simulink model "control_pos_6dof_conMI"  (R2023b)
settings: Solver=ode45  StartTime=0.0  StopTime=tsim  FixedStep=tstep  MaxStep=tstep
undefined symbols (not defined in the file): a0, a1, MI_Contr1, MI_Contr2, MI_Contr3, MI_Contr4, MI_Contr5, MI_Contr6, MI_motor1, MI_motor2, MI_motor3, MI_motor4, MI_motor5, MI_motor6, robot_params, sigbuilder_block, t_qeq_init, t_tr_init, tau_L, tr_ref
(part 6 of 10)

== matlab function control_pos_6dof_conMI/Controlador/Modelo dinámico ==
  data: robot_params input; robot_din output Bus: robot_din_bus size=1; q input size=[6,1]; dq input size=[6,1]
function robot_din = fcn(robot_params,q,dq)


% l1 = robot_params.l(1);
l2 = robot_params.l(2);
l3 = robot_params.l(3);
% l4 = robot_params.l(4);
% l5 = robot_params.l(5);
% l6 = robot_params.l(6);

lc1 = robot_params.lc(1);
lc2 = robot_params.lc(2);
lc3 = robot_params.lc(3);
% lc4 = robot_params.lc(4);
% lc5 = robot_params.lc(5);
% lc6 = robot_params.lc(6);

d1 = robot_params.d(1);
d2 = robot_params.d(2);
d3 = robot_params.d(3);
d4 = robot_params.d(4);
d5 = robot_params.d(5);
d6 = robot_params.d(6);

% dc1 = robot_params.dc(1);
% dc2 = robot_params.dc(2);
% dc3 = robot_params.dc(3);
dc4 = robot_params.dc(4);
dc5 = robot_params.dc(5);
dc6 = robot_params.dc(6);

m1 = robot_params.m(1);
m2 = robot_params.m(2);
m3 = robot_params.m(3);
m4 = robot_params.m(4);
m5 = robot_params.m(5);
m6 = robot_params.m(6);

%Posiciones angulares
% q1 = q(1);
q2 = q(2);
q3 = q(3);
q4 = q(4);
q5 = q(5);
% q6 = q(6);

%Velocidades angulares
dq1 = dq(1);
dq2 = dq(2);
dq3 = dq(3);
dq4 = dq(4);
dq5 = dq(5);
% dq6 = dq(6);

% Matriz de Inercia D
D = zeros(6,6);

D(1,1) = (d1*m1)/2 + (d2*m2)/2 + (d3*m3)/2 + (d4*m4)/2 + (d5*m5)/2 + (d6*m6)/2 + d4^2*m5 + d4^2*m6 + (d5^2*m6)/2 + dc4^2*m4 + (dc5^2*m5)/2 + (3*dc6^2*m6)/4 + (l2^2*m3)/2 + (l2^2*m4)/2 + (l2^2*m5)/2 + (l3^2*m4)/2 + (l2^2*m6)/2 + (l3^2*m5)/2 + (l3^2*m6)/2 + lc1^2*m1 + (lc2^2*m2)/2 + (lc3^2*m3)/2 - (dc6^2*m6*cos(2*q2 + 2*q3 + 2*q4 - 2*q5))/8 - (dc6^2*m6*cos(2*q2 + 2*q3 + 2*q4 + 2*q5))/8 - (d5^2*m6*cos(2*q2 + 2*q3 + 2*q4))/2 + (dc6^2*m6*cos(2*q5))/4 - (dc5^2*m5*cos(2*q2 + 2*q3 + 2*q4))/2 + (dc6^2*m6*cos(2*q2 + 2*q3 + 2*q4))/4 + (l2^2*m3*cos(2*q2))/2 + (l2^2*m4*cos(2*q2))/2 + (l2^2*m5*cos(2*q2))/2 + (l2^2*m6*cos(2*q2))/2 + (lc2^2*m2*cos(2*q2))/2 + (l3^2*m4*cos(2*q2 + 2*q3))/2 + (l3^2*m5*cos(2*q2 + 2*q3))/2 + (l3^2*m6*cos(2*q2 + 2*q3))/2 + (lc3^2*m3*cos(2*q2 + 2*q3))/2 + d5*l2*m6*sin(2*q2 + q3 + q4) + dc5*l2*m5*sin(2*q2 + q3 + q4) + (dc6*l2*m6*sin(q3 + q4 - q5))/2 + (d5*dc6*m6*cos(2*q2 + 2*q3 + 2*q4 + q5))/2 + d5*l2*m6*sin(q3 + q4) + dc5*l2*m5*sin(q3 + q4) - (dc6*l3*m6*sin(q4 + q5))/2 + (dc6*l3*m6*sin(2*q2 + 2*q3 + q4 - q5))/2 + 2*d4*dc6*m6*cos(q5) + l2*l3*m4*cos(q3) + l2*l3*m5*cos(q3) + l2*l3*m6*cos(q3) + l2*lc3*m3*cos(q3) + d5*l3*m6*sin(q4) + d5*l3*m6*sin(2*q2 + 2*q3 + q4) + dc5*l3*m5*sin(q4) + dc5*l3*m5*sin(2*q2 + 2*q3 + q4) - (dc6*l2*m6*sin(2*q2 + q3 + q4 + q5))/2 - (d5*dc6*m6*cos(2*q2 + 2*q3 + 2*q4 - q5))/2 + l2*l3*m4*cos(2*q2 + q3) + l2*l3*m5*cos(2*q2 + q3) + l2*l3*m6*cos(2*q2 + q3) + l2*lc3*m3*cos(2*q2 + q3) + (dc6*l3*m6*sin(q4 - q5))/2 - (dc6*l2*m6*sin(q3 + q4 + q5))/2 + (dc6*l2*m6*sin(2*q2 + q3 + q4 - q5))/2 - (dc6*l3*m6*sin(2*q2 + 2*q3 + q4 + q5))/2;
D(1,2) = (dc6^2*m6*cos(q2 + q3 + q4 - 2*q5))/4 - (dc6^2*m6*cos(q2 + q3 + q4 + 2*q5))/4 - (d4*dc6*m6*cos(q2 + q3 + q4 + q5))/2 + (d5*dc6*m6*cos(q2 + q3 + q4 + q5))/2 - (dc6*l3*m6*sin(q2 + q3 - q5))/2 - d4*l3*m5*sin(q2 + q3) - d4*l3*m6*sin(q2 + q3) - dc4*l3*m4*sin(q2 + q3) - (dc6*l2*m6*sin(q2 + q5))/2 + (d4*dc6*m6*cos(q2 + q3 + q4 - q5))/2 + (d5*dc6*m6*cos(q2 + q3 + q4 - q5))/2 - d4*l2*m5*sin(q2) - d4*l2*m6*sin(q2) - dc4*l2*m4*sin(q2) + d4*d5*m6*cos(q2 + q3 + q4) + d4*dc5*m5*cos(q2 + q3 + q4) - (dc6*l2*m6*sin(q2 - q5))/2 - (dc6*l3*m6*sin(q2 + q3 + q5))/2;
D(1,3) = (dc6^2*m6*cos(q2 + q3 + q4 - 2*q5))/4 - (dc6^2*m6*cos(q2 + q3 + q4 + 2*q5))/4 - (d4*dc6*m6*cos(q2 + q3 + q4 + q5))/2 + (d5*dc6*m6*cos(q2 + q3 + q4 + q5))/2 - (dc6*l3*m6*sin(q2 + q3 - q5))/2 - d4*l3*m5*sin(q2 + q3) - d4*l3*m6*sin(q2 + q3) - dc4*l3*m4*sin(q2 + q3) + (d4*dc6*m6*cos(q2 + q3 + q4 - q5))/2 + (d5*dc6*m6*cos(q2 + q3 + q4 - q5))/2 + d4*d5*m6*cos(q2 + q3 + q4) + d4*dc5*m5*cos(q2 + q3 + q4) - (dc6*l3*m6*sin(q2 + q3 + q5))/2;
D(1,4) = (dc6^2*m6*cos(q2 + q3 + q4 - 2*q5))/4 - (dc6^2*m6*cos(q2 + q3 + q4 + 2*q5))/4 - (d4*dc6*m6*cos(q2 + q3 + q4 + q5))/2 + (d5*dc6*m6*cos(q2 + q3 + q4 + q5))/2 + (d4*dc6*m6*cos(q2 + q3 + q4 - q5))/2 + (d5*dc6*m6*cos(q2 + q3 + q4 - q5))/2 + d4*d5*m6*cos(q2 + q3 + q4) + d4*dc5*m5*cos(q2 + q3 + q4);
D(1,5) = -(dc6*m6*(d4*cos(q2 + q3 + q4 + q5) + d5*cos(q2 + q3 + q4 + q5) + l3*sin(q2 + q3 - q5) - l2*sin(q2 + q5) + d4*cos(q2 + q3 + q4 - q5) - d5*cos(q2 + q3 + q4 - q5) + 2*dc6*cos(q2 + q3 + q4) + l2*sin(q2 - q5) - l3*sin(q2 + q3 + q5)))/2;
D(1,6) = 0;

D(2,1) = (dc6^2*m6*cos(q2 + q3 + q4 - 2*q5))/4 - (dc6^2*m6*cos(q2 + q3 + q4 + 2*q5))/4 - (d4*dc6*m6*cos(q2 + q3 + q4 + q5))/2 + (d5*dc6*m6*cos(q2 + q3 + q4 + q5))/2 - (dc6*l3*m6*sin(q2 + q3 - q5))/2 - d4*l3*m5*sin(q2 + q3) - d4*l3*m6*sin(q2 + q3) - dc4*l3*m4*sin(q2 + q3) - (dc6*l2*m6*sin(q2 + q5))/2 + (d4*dc6*m6*cos(q2 + q3 + q4 - q5))/2 + (d5*dc6*m6*cos(q2 + q3 + q4 - q5))/2 - d4*l2*m5*sin(q2) - d4*l2*m6*sin(q2) - dc4*l2*m4*sin(q2) + d4*d5*m6*cos(q2 + q3 + q4) + d4*dc5*m5*cos(q2 + q3 + q4) - (dc6*l2*m6*sin(q2 - q5))/2 - (dc6*l3*m6*sin(q2 + q3 + q5))/2;
D(2,2) = (d2*m2)/2 + (d3*m3)/2 + (d4*m4)/2 + (d5*m5)/2 + (d6*m6)/2 + d5^2*m6 + dc5^2*m5 + (dc6^2*m6)/2 + l2^2*m3 + l2^2*m4 + l2^2*m5 + l3^2*m4 + l2^2*m6 + l3^2*m5 + l3^2*m6 + lc2^2*m2 + lc3^2*m3 - (dc6^2*m6*cos(2*q5))/2 + 2*d5*l2*m6*sin(q3 + q4) + 2*dc5*l2*m5*sin(q3 + q4) + 2*l2*l3*m4*cos(q3) + 2*l2*l3*m5*cos(q3) + 2*l2*l3*m6*cos(q3) + 2*l2*lc3*m3*cos(q3) + 2*d5*l3*m6*sin(q4) + 2*dc5*l3*m5*sin(q4) - 2*dc6*l3*m6*cos(q4)*sin(q5) - 2*dc6*l2*m6*cos(q3)*cos(q4)*sin(q5) + 2*dc6*l2*m6*sin(q3)*sin(q4)*sin(q5);
D(2,3) = d5^2*m6 + dc5^2*m5 + (dc6^2*m6)/2 + l3^2*m4 + l3^2*m5 + l3^2*m6 + lc3^2*m3 - (dc6^2*m6*cos(2*q5))/2 + d5*l2*m6*sin(q3 + q4) + dc5*l2*m5*sin(q3 + q4) + l2*l3*m4*cos(q3) + l2*l3*m5*cos(q3) + l2*l3*m6*cos(q3) + l2*lc3*m3*cos(q3) + 2*d5*l3*m6*sin(q4) + 2*dc5*l3*m5*sin(q4) - 2*dc6*l3*m6*cos(q4)*sin(q5) - dc6*l2*m6*cos(q3)*cos(q4)*sin(q5) + dc6*l2*m6*sin(q3)*sin(q4)*sin(q5);
D(2,4) = d5^2*m6 + dc5^2*m5 + (dc6^2*m6)/2 - (dc6^2*m6*cos(2*q5))/2 + d5*l2*m6*sin(q3 + q4) + dc5*l2*m5*sin(q3 + q4) + d5*l3*m6*sin(q4) + dc5*l3*m5*sin(q4) - dc6*l3*m6*cos(q4)*sin(q5) - dc6*l2*m6*cos(q3)*cos(q4)*sin(q5) + dc6*l2*m6*sin(q3)*sin(q4)*sin(q5);
D(2,5) = -dc6*m6*cos(q5)*(d5 + l2*sin(q3 + q4) + l3*sin(q4));
D(2,6) = 0;

D(3,1) = (dc6^2*m6*cos(q2 + q3 + q4 - 2*q5))/4 - (dc6^2*m6*cos(q2 + q3 + q4 + 2*q5))/4 - (d4*dc6*m6*cos(q2 + q3 + q4 + q5))/2 + (d5*dc6*m6*cos(q2 + q3 + q4 + q5))/2 - (dc6*l3*m6*sin(q2 + q3 - q5))/2 - d4*l3*m5*sin(q2 + q3) - d4*l3*m6*sin(q2 + q3) - dc4*l3*m4*sin(q2 + q3) + (d4*dc6*m6*cos(q2 + q3 + q4 - q5))/2 + (d5*dc6*m6*cos(q2 + q3 + q4 - q5))/2 + d4*d5*m6*cos(q2 + q3 + q4) + d4*dc5*m5*cos(q2 + q3 + q4) - (dc6*l3*m6*sin(q2 + q3 + q5))/2;
D(3,2) = d5^2*m6 + dc5^2*m5 + (dc6^2*m6)/2 + l3^2*m4 + l3^2*m5 + l3^2*m6 + lc3^2*m3 - (dc6^2*m6*cos(2*q5))/2 + d5*l2*m6*sin(q3 + q4) + dc5*l2*m5*sin(q3 + q4) + l2*l3*m4*cos(q3) + l2*l3*m5*cos(q3) + l2*l3*m6*cos(q3) + l2*lc3*m3*cos(q3) + 2*d5*l3*m6*sin(q4) + 2*dc5*l3*m5*sin(q4) - 2*dc6*l3*m6*cos(q4)*sin(q5) - dc6*l2*m6*cos(q3)*cos(q4)*sin(q5) + dc6*l2*m6*sin(q3)*sin(q4)*sin(q5);
D(3,3) = (d3*m3)/2 + (d4*m4)/2 + (d5*m5)/2 + (d6*m6)/2 + d5^2*m6 + dc5^2*m5 + l3^2*m4 + l3^2*m5 + l3^2*m6 + lc3^2*m3 + dc6^2*m6*sin(q5)^2 + 2*d5*l3*m6*sin(q4) + 2*dc5*l3*m5*sin(q4) - 2*dc6*l3*m6*cos(q4)*sin(q5);
D(3,4) = d5^2*m6 + dc5^2*m5 + dc6^2*m6*sin(q5)^2 + d5*l3*m6*sin(q4) + dc5*l3*m5*sin(q4) - dc6*l3*m6*cos(q4)*sin(q5);
D(3,5) = -dc6*m6*cos(q5)*(d5 + l3*sin(q4));
D(3,6) = 0;

D(4,1) = (dc6^2*m6*cos(q2 + q3 + q4 - 2*q5))/4 - (dc6^2*m6*cos(q2 + q3 + q4 + 2*q5))/4 - (d4*dc6*m6*cos(q2 + q3 + q4 + q5))/2 + (d5*dc6*m6*cos(q2 + q3 + q4 + q5))/2 + (d4*dc6*m6*cos(q2 + q3 + q4 - q5))/2 + (d5*dc6*m6*cos(q2 + q3 + q4 - q5))/2 + d4*d5*m6*cos(q2 + q3 + q4) + d4*dc5*m5*cos(q2 + q3 + q4);
D(4,2) = d5^2*m6 + dc5^2*m5 + (dc6^2*m6)/2 - (dc6^2*m6*cos(2*q5))/2 + d5*l2*m6*sin(q3 + q4) + dc5*l2*m5*sin(q3 + q4) + d5*l3*m6*sin(q4) + dc5*l3*m5*sin(q4) - dc6*l3*m6*cos(q4)*sin(q5) - dc6*l2*m6*cos(q3)*cos(q4)*sin(q5) + dc6*l2*m6*sin(q3)*sin(q4)*sin(q5);
D(4,3) = d5^2*m6 + dc5^2*m5 + dc6^2*m6*sin(q5)^2 + d5*l3*m6*sin(q4) + dc5*l3*m5*sin(q4) - dc6*l3*m6*cos(q4)*sin(q5);
D(4,4) = (d4*m4)/2 + (d5*m5)/2 + (d6*m6)/2 + d5^2*m6 + dc5^2*m5 + dc6^2*m6 - dc6^2*m6*cos(q5)^2;
D(4,5) = -d5*dc6*m6*cos(q5);
D(4,6) = 0;

D(5,1) = -(dc6*m6*(d4*cos(q2 + q3 + q4 + q5) + d5*cos(q2 + q3 + q4 + q5) + l3*sin(q2 + q3 - q5) - l2*sin(q2 + q5) + d4*cos(q2 + q3 + q4 - q5) - d5*cos(q2 + q3 + q4 - q5) + 2*dc6*cos(q2 + q3 + q4) + l2*sin(q2 - q5) - l3*sin(q2 + q3 + q5)))/2;
D(5,2) = -dc6*m6*cos(q5)*(d5 + l2*sin(q3 + q4) + l3*sin(q4));
D(5,3) = -dc6*m6*cos(q5)*(d5 + l3*sin(q4));
D(5,4) = -d5*dc6*m6*cos(q5);
D(5,5) = (d5*m5)/2 + (d6*m6)/2 + dc6^2*m6;
D(5,6) = 0;

D(6,1) = 0;
D(6,2) = 0;
D(6,3) = 0;
D(6,4) = 0;
D(6,5) = 0;
D(6,6) = 1;

% Matriz de Coriollis C
C = zeros(6,6);

C(1,1) = 0;
C(1,2) = (dc6^2*dq1*m6*sin(2*q2 + 2*q3 + 2*q4 - 2*q5))/4 + (dc6^2*dq1*m6*sin(2*q2 + 2*q3 + 2*q4 + 2*q5))/4 + d5^2*dq1*m6*sin(2*q2 + 2*q3 + 2*q4) + dc5^2*dq1*m5*sin(2*q2 + 2*q3 + 2*q4) - (dc6^2*dq1*m6*sin(2*q2 + 2*q3 + 2*q4))/2 - dq1*l2^2*m3*sin(2*q2) - dq1*l2^2*m4*sin(2*q2) - dq1*l2^2*m5*sin(2*q2) - dq1*l2^2*m6*sin(2*q2) - dq1*lc2^2*m2*sin(2*q2) - dq1*l3^2*m4*sin(2*q2 + 2*q3) - dq1*l3^2*m5*sin(2*q2 + 2*q3) - dq1*l3^2*m6*sin(2*q2 + 2*q3) - dq1*lc3^2*m3*sin(2*q2 + 2*q3) - (dc6^2*dq2*m6*sin(q2 + q3 + q4 - 2*q5))/4 + (dc6^2*dq2*m6*sin(q2 + q3 + q4 + 2*q5))/4 - (dc6*dq2*l2*m6*cos(q2 - q5))/2 + d5*dc6*dq1*m6*sin(2*q2 + 2*q3 + 2*q4 - q5) - (dc6*dq2*l3*m6*cos(q2 + q3 + q5))/2 - 2*dq1*l2*l3*m4*sin(2*q2 + q3) - 2*dq1*l2*l3*m5*sin(2*q2 + q3) - 2*dq1*l2*l3*m6*sin(2*q2 + q3) - 2*dq1*l2*lc3*m3*sin(2*q2 + q3) - d4*d5*dq2*m6*sin(q2 + q3 + q4) - d4*dc5*dq2*m5*sin(q2 + q3 + q4) + dc6*dq1*l2*m6*cos(2*q2 + q3 + q4 - q5) - dc6*dq1*l3*m6*cos(2*q2 + 2*q3 + q4 + q5) + 2*d5*dq1*l2*m6*cos(2*q2 + q3 + q4) + 2*dc5*dq1*l2*m5*cos(2*q2 + q3 + q4) - (dc6*dq2*l3*m6*cos(q2 + q3 - q5))/2 + (d4*dc6*dq2*m6*sin(q2 + q3 + q4 + q5))/2 - (d5*dc6*dq2*m6*sin(q2 + q3 + q4 + q5))/2 - d4*dq2*l3*m5*cos(q2 + q3) - d4*dq2*l3*m6*cos(q2 + q3) - dc4*dq2*l3*m4*cos(q2 + q3) - (dc6*dq2*l2*m6*cos(q2 + q5))/2 + dc6*dq1*l3*m6*cos(2*q2 + 2*q3 + q4 - q5) - d5*dc6*dq1*m6*sin(2*q2 + 2*q3 + 2*q4 + q5) - d4*dq2*l2*m5*cos(q2) - d4*dq2*l2*m6*cos(q2) + 2*d5*dq1*l3*m6*cos(2*q2 + 2*q3 + q4) - dc4*dq2*l2*m4*cos(q2) + 2*dc5*dq1*l3*m5*cos(2*q2 + 2*q3 + q4) - dc6*dq1*l2*m6*cos(2*q2 + q3 + q4 + q5) - (d4*dc6*dq2*m6*sin(q2 + q3 + q4 - q5))/2 - (d5*dc6*dq2*m6*sin(q2 + q3 + q4 - q5))/2;
C(1,3) = (dc6^2*dq1*m6*sin(2*q2 + 2*q3 + 2*q4 - 2*q5))/4 + (dc6^2*dq1*m6*sin(2*q2 + 2*q3 + 2*q4 + 2*q5))/4 + d5^2*dq1*m6*sin(2*q2 + 2*q3 + 2*q4) + dc5^2*dq1*m5*sin(2*q2 + 2*q3 + 2*q4) - (dc6^2*dq1*m6*sin(2*q2 + 2*q3 + 2*q4))/2 - dq1*l3^2*m4*sin(2*q2 + 2*q3) - dq1*l3^2*m5*sin(2*q2 + 2*q3) - dq1*l3^2*m6*sin(2*q2 + 2*q3) - dq1*lc3^2*m3*sin(2*q2 + 2*q3) - (dc6^2*dq2*m6*sin(q2 + q3 + q4 - 2*q5))/2 + (dc6^2*dq2*m6*sin(q2 + q3 + q4 + 2*q5))/2 - (dc6^2*dq3*m6*sin(q2 + q3 + q4 - 2*q5))/4 + (dc6^2*dq3*m6*sin(q2 + q3 + q4 + 2*q5))/4 + d5*dc6*dq1*m6*sin(2*q2 + 2*q3 + 2*q4 - q5) - (dc6*dq1*l2*m6*cos(q3 + q4 + q5))/2 - dc6*dq2*l3*m6*cos(q2 + q3 + q5) - (dc6*dq3*l3*m6*cos(q2 + q3 + q5))/2 - dq1*l2*l3*m4*sin(2*q2 + q3) - dq1*l2*l3*m5*sin(2*q2 + q3) - dq1*l2*l3*m6*sin(2*q2 + q3) - dq1*l2*lc3*m3*sin(2*q2 + q3) - 2*d4*d5*dq2*m6*sin(q2 + q3 + q4) - d4*d5*dq3*m6*sin(q2 + q3 + q4) - 2*d4*dc5*dq2*m5*sin(q2 + q3 + q4) - d4*dc5*dq3*m5*sin(q2 + q3 + q4) + (dc6*dq1*l2*m6*cos(2*q2 + q3 + q4 - q5))/2 - dc6*dq1*l3*m6*cos(2*q2 + 2*q3 + q4 + q5) + d5*dq1*l2*m6*cos(2*q2 + q3 + q4) + dc5*dq1*l2*m5*cos(2*q2 + q3 + q4) + (dc6*dq1*l2*m6*cos(q3 + q4 - q5))/2 - dc6*dq2*l3*m6*cos(q2 + q3 - q5) - (dc6*dq3*l3*m6*cos(q2 + q3 - q5))/2 + d4*dc6*dq2*m6*sin(q2 + q3 + q4 + q5) + (d4*dc6*dq3*m6*sin(q2 + q3 + q4 + q5))/2 - d5*dc6*dq2*m6*sin(q2 + q3 + q4 + q5) - (d5*dc6*dq3*m6*sin(q2 + q3 + q4 + q5))/2 - 2*d4*dq2*l3*m5*cos(q2 + q3) - 2*d4*dq2*l3*m6*cos(q2 + q3) - d4*dq3*l3*m5*cos(q2 + q3) - d4*dq3*l3*m6*cos(q2 + q3) + d5*dq1*l2*m6*cos(q3 + q4) - 2*dc4*dq2*l3*m4*cos(q2 + q3) - dc4*dq3*l3*m4*cos(q2 + q3) + dc5*dq1*l2*m5*cos(q3 + q4) + dc6*dq1*l3*m6*cos(2*q2 + 2*q3 + q4 - q5) - d5*dc6*dq1*m6*sin(2*q2 + 2*q3 + 2*q4 + q5) + 2*d5*dq1*l3*m6*cos(2*q2 + 2*q3 + q4) + 2*dc5*dq1*l3*m5*cos(2*q2 + 2*q3 + q4) - (dc6*dq1*l2*m6*cos(2*q2 + q3 + q4 + q5))/2 - dq1*l2*l3*m4*sin(q3) - dq1*l2*l3*m5*sin(q3) - dq1*l2*l3*m6*sin(q3) - dq1*l2*lc3*m3*sin(q3) - d4*dc6*dq2*m6*sin(q2 + q3 + q4 - q5) - (d4*dc6*dq3*m6*sin(q2 + q3 + q4 - q5))/2 - d5*dc6*dq2*m6*sin(q2 + q3 + q4 - q5) - (d5*dc6*dq3*m6*sin(q2 + q3 + q4 - q5))/2;
C(1,4) = (dc6^2*dq1*m6*sin(2*q2 + 2*q3 + 2*q4 - 2*q5))/4 + (dc6^2*dq1*m6*sin(2*q2 + 2*q3 + 2*q4 + 2*q5))/4 + d5^2*dq1*m6*sin(2*q2 + 2*q3 + 2*q4) + dc5^2*dq1*m5*sin(2*q2 + 2*q3 + 2*q4) - (dc6^2*dq1*m6*sin(2*q2 + 2*q3 + 2*q4))/2 - (dc6^2*dq2*m6*sin(q2 + q3 + q4 - 2*q5))/2 + (dc6^2*dq2*m6*sin(q2 + q3 + q4 + 2*q5))/2 - (dc6^2*dq3*m6*sin(q2 + q3 + q4 - 2*q5))/2 + (dc6^2*dq3*m6*sin(q2 + q3 + q4 + 2*q5))/2 - (dc6^2*dq4*m6*sin(q2 + q3 + q4 - 2*q5))/4 + (dc6^2*dq4*m6*sin(q2 + q3 + q4 + 2*q5))/4 + (dc6*dq1*l3*m6*cos(q4 - q5))/2 + d5*dc6*dq1*m6*sin(2*q2 + 2*q3 + 2*q4 - q5) - (dc6*dq1*l2*m6*cos(q3 + q4 + q5))/2 - 2*d4*d5*dq2*m6*sin(q2 + q3 + q4) - 2*d4*d5*dq3*m6*sin(q2 + q3 + q4) - d4*d5*dq4*m6*sin(q2 + q3 + q4) - 2*d4*dc5*dq2*m5*sin(q2 + q3 + q4) - 2*d4*dc5*dq3*m5*sin(q2 + q3 + q4) - d4*dc5*dq4*m5*sin(q2 + q3 + q4) + (dc6*dq1*l2*m6*cos(2*q2 + q3 + q4 - q5))/2 - (dc6*dq1*l3*m6*cos(2*q2 + 2*q3 + q4 + q5))/2 + d5*dq1*l2*m6*cos(2*q2 + q3 + q4) + dc5*dq1*l2*m5*cos(2*q2 + q3 + q4) + (dc6*dq1*l2*m6*cos(q3 + q4 - q5))/2 + d4*dc6*dq2*m6*sin(q2 + q3 + q4 + q5) + d4*dc6*dq3*m6*sin(q2 + q3 + q4 + q5) - d5*dc6*dq2*m6*sin(q2 + q3 + q4 + q5) + (d4*dc6*dq4*m6*sin(q2 + q3 + q4 + q5))/2 - d5*dc6*dq3*m6*sin(q2 + q3 + q4 + q5) - (d5*dc6*dq4*m6*sin(q2 + q3 + q4 + q5))/2 + d5*dq1*l2*m6*cos(q3 + q4) + dc5*dq1*l2*m5*cos(q3 + q4) - (dc6*dq1*l3*m6*cos(q4 + q5))/2 + (dc6*dq1*l3*m6*cos(2*q2 + 2*q3 + q4 - q5))/2 - d5*dc6*dq1*m6*sin(2*q2 + 2*q3 + 2*q4 + q5) + d5*dq1*l3*m6*cos(q4) + d5*dq1*l3*m6*cos(2*q2 + 2*q3 + q4) + dc5*dq1*l3*m5*cos(q4) + dc5*dq1*l3*m5*cos(2*q2 + 2*q3 + q4) - (dc6*dq1*l2*m6*cos(2*q2 + q3 + q4 + q5))/2 - d4*dc6*dq2*m6*sin(q2 + q3 + q4 - q5) - d4*dc6*dq3*m6*sin(q2 + q3 + q4 - q5) - d5*dc6*dq2*m6*sin(q2 + q3 + q4 - q5) - (d4*dc6*dq4*m6*sin(q2 + q3 + q4 - q5))/2 - d5*dc6*dq3*m6*sin(q2 + q3 + q4 - q5) - (d5*dc6*dq4*m6*sin(q2 + q3 + q4 - q5))/2;
C(1,5) = (dc6*m6*(4*d4*dq2*sin(q2 + q3 + q4 - q5) - 2*dq1*l2*cos(2*q2 + q3 + q4 + q5) - 8*d4*dq1*sin(q5) + 4*d4*dq3*sin(q2 + q3 + q4 - q5) + 4*d4*dq4*sin(q2 + q3 + q4 - q5) - 2*d4*dq5*sin(q2 + q3 + q4 - q5) + 2*d5*dq5*sin(q2 + q3 + q4 - q5) + 2*dc6*dq2*sin(q2 + q3 + q4 - 2*q5) + 2*dc6*dq2*sin(q2 + q3 + q4 + 2*q5) + 2*dc6*dq3*sin(q2 + q3 + q4 - 2*q5) + 2*dc6*dq3*sin(q2 + q3 + q4 + 2*q5) + 2*dc6*dq4*sin(q2 + q3 + q4 - 2*q5) + 2*dc6*dq4*sin(q2 + q3 + q4 + 2*q5) - 2*dq1*l3*cos(q4 - q5) + 2*dq5*l2*cos(q2 - q5) - 2*d5*dq1*sin(2*q2 + 2*q3 + 2*q4 - q5) - dc6*dq1*sin(2*q2 + 2*q3 + 2*q4 - 2*q5) + dc6*dq1*sin(2*q2 + 2*q3 + 2*q4 + 2*q5) - 2*dq1*l2*cos(q3 + q4 + q5) + 2*dq5*l3*cos(q2 + q3 + q5) + 4*dc6*dq2*sin(q2 + q3 + q4) + 4*dc6*dq3*sin(q2 + q3 + q4) + 4*dc6*dq4*sin(q2 + q3 + q4) - 2*dc6*dq1*sin(2*q5) - 2*dq1*l2*cos(2*q2 + q3 + q4 - q5) - 2*dq1*l3*cos(2*q2 + 2*q3 + q4 + q5) - 2*dq1*l2*cos(q3 + q4 - q5) + 2*dq5*l3*cos(q2 + q3 - q5) + 4*d4*dq2*sin(q2 + q3 + q4 + q5) + 4*d4*dq3*sin(q2 + q3 + q4 + q5) + 4*d4*dq4*sin(q2 + q3 + q4 + q5) + 2*d4*dq5*sin(q2 + q3 + q4 + q5) + 2*d5*dq5*sin(q2 + q3 + q4 + q5) - 2*dq1*l3*cos(q4 + q5) + 2*dq5*l2*cos(q2 + q5) - 2*dq1*l3*cos(2*q2 + 2*q3 + q4 - q5) - 2*d5*dq1*sin(2*q2 + 2*q3 + 2*q4 + q5)))/4;
C(1,6) = 0;

C(2,1) = (dc6^2*dq1*m6*sin(2*q2 + 2*q3 + 2*q4))/4 - (dc6^2*dq1*m6*sin(2*q2 + 2*q3 + 2*q4 + 2*q5))/8 - (d5^2*dq1*m6*sin(2*q2 + 2*q3 + 2*q4))/2 - (dc5^2*dq1*m5*sin(2*q2 + 2*q3 + 2*q4))/2 - (dc6^2*dq1*m6*sin(2*q2 + 2*q3 + 2*q4 - 2*q5))/8 + (dq1*l2^2*m3*sin(2*q2))/2 + (dq1*l2^2*m4*sin(2*q2))/2 + (dq1*l2^2*m5*sin(2*q2))/2 + (dq1*l2^2*m6*sin(2*q2))/2 + (dq1*lc2^2*m2*sin(2*q2))/2 + (dq1*l3^2*m4*sin(2*q2 + 2*q3))/2 + (dq1*l3^2*m5*sin(2*q2 + 2*q3))/2 + (dq1*l3^2*m6*sin(2*q2 + 2*q3))/2 + (dq1*lc3^2*m3*sin(2*q2 + 2*q3))/2 - (d5*dc6*dq1*m6*sin(2*q2 + 2*q3 + 2*q4 - q5))/2 + dq1*l2*l3*m4*sin(2*q2 + q3) + dq1*l2*l3*m5*sin(2*q2 + q3) + dq1*l2*l3*m6*sin(2*q2 + q3) + dq1*l2*lc3*m3*sin(2*q2 + q3) - (dc6*dq1*l2*m6*cos(2*q2 + q3 + q4 - q5))/2 + (dc6*dq1*l3*m6*cos(2*q2 + 2*q3 + q4 + q5))/2 - d5*dq1*l2*m6*cos(2*q2 + q3 + q4) - dc5*dq1*l2*m5*cos(2*q2 + q3 + q4) - (dc6*dq1*l3*m6*cos(2*q2 + 2*q3 + q4 - q5))/2 + (d5*dc6*dq1*m6*sin(2*q2 + 2*q3 + 2*q4 + q5))/2 - d5*dq1*l3*m6*cos(2*q2 + 2*q3 + q4) - dc5*dq1*l3*m5*cos(2*q2 + 2*q3 + q4) + (dc6*dq1*l2*m6*cos(2*q2 + q3 + q4 + q5))/2;
C(2,2) = 0;
C(2,3) = -l2*(2*dq2 + dq3)*(l3*m4*sin(q3) + l3*m5*sin(q3) + l3*m6*sin(q3) + lc3*m3*sin(q3) - d5*m6*cos(q3 + q4) - dc5*m5*cos(q3 + q4) - dc6*m6*cos(q3)*sin(q4)*sin(q5) - dc6*m6*cos(q4)*sin(q3)*sin(q5));
C(2,4) = (dc6*dq4*l3*m6*cos(q4 - q5))/2 + 2*d5*dq2*l2*m6*cos(q3 + q4) + 2*d5*dq3*l2*m6*cos(q3 + q4) + d5*dq4*l2*m6*cos(q3 + q4) + 2*dc5*dq2*l2*m5*cos(q3 + q4) + 2*dc5*dq3*l2*m5*cos(q3 + q4) + dc5*dq4*l2*m5*cos(q3 + q4) - (dc6*dq4*l3*m6*cos(q4 + q5))/2 + 2*d5*dq2*l3*m6*cos(q4) + 2*d5*dq3*l3*m6*cos(q4) + d5*dq4*l3*m6*cos(q4) + 2*dc5*dq2*l3*m5*cos(q4) + 2*dc5*dq3*l3*m5*cos(q4) + dc5*dq4*l3*m5*cos(q4) + 2*dc6*dq2*l3*m6*sin(q4)*sin(q5) + 2*dc6*dq3*l3*m6*sin(q4)*sin(q5) + 2*dc6*dq2*l2*m6*cos(q3)*sin(q4)*sin(q5) + 2*dc6*dq2*l2*m6*cos(q4)*sin(q3)*sin(q5) + 2*dc6*dq3*l2*m6*cos(q3)*sin(q4)*sin(q5) + 2*dc6*dq3*l2*m6*cos(q4)*sin(q3)*sin(q5) + dc6*dq4*l2*m6*cos(q3)*sin(q4)*sin(q5) + dc6*dq4*l2*m6*cos(q4)*sin(q3)*sin(q5);
C(2,5) = -(dc6*m6*(2*dq2*l3*cos(q4 - q5) - 2*d5*dq1*sin(q2 + q3 + q4 - q5) - dc6*dq1*sin(q2 + q3 + q4 - 2*q5) - dc6*dq1*sin(q2 + q3 + q4 + 2*q5) - 2*dq1*l2*cos(q2 - q5) - 2*d5*dq5*sin(q5) + 2*dq3*l3*cos(q4 - q5) + 2*dq4*l3*cos(q4 - q5) - dq5*l3*cos(q4 - q5) + 2*dq1*l3*cos(q2 + q3 + q5) + 2*dq2*l2*cos(q3 + q4 + q5) + 2*dq3*l2*cos(q3 + q4 + q5) + 2*dq4*l2*cos(q3 + q4 + q5) + dq5*l2*cos(q3 + q4 + q5) + 2*dc6*dq1*sin(q2 + q3 + q4) - 2*dc6*dq2*sin(2*q5) - 2*dc6*dq3*sin(2*q5) - 2*dc6*dq4*sin(2*q5) - 2*dq1*l3*cos(q2 + q3 - q5) + 2*dq2*l2*cos(q3 + q4 - q5) + 2*dq3*l2*cos(q3 + q4 - q5) + 2*dq4*l2*cos(q3 + q4 - q5) - dq5*l2*cos(q3 + q4 - q5) + 2*d5*dq1*sin(q2 + q3 + q4 + q5) + 2*dq1*l2*cos(q2 + q5) + 2*dq2*l3*cos(q4 + q5) + 2*dq3*l3*cos(q4 + q5) + 2*dq4*l3*cos(q4 + q5) + dq5*l3*cos(q4 + q5)))/2;
C(2,6) = 0;

C(3,1) = (dc6^2*dq1*m6*sin(2*q2 + 2*q3 + 2*q4))/4 - (dc6^2*dq1*m6*sin(2*q2 + 2*q3 + 2*q4 + 2*q5))/8 - (d5^2*dq1*m6*sin(2*q2 + 2*q3 + 2*q4))/2 - (dc5^2*dq1*m5*sin(2*q2 + 2*q3 + 2*q4))/2 - (dc6^2*dq1*m6*sin(2*q2 + 2*q3 + 2*q4 - 2*q5))/8 + (dq1*l3^2*m4*sin(2*q2 + 2*q3))/2 + (dq1*l3^2*m5*sin(2*q2 + 2*q3))/2 + (dq1*l3^2*m6*sin(2*q2 + 2*q3))/2 + (dq1*lc3^2*m3*sin(2*q2 + 2*q3))/2 - (d5*dc6*dq1*m6*sin(2*q2 + 2*q3 + 2*q4 - q5))/2 + (dc6*dq1*l2*m6*cos(q3 + q4 + q5))/4 + (dq1*l2*l3*m4*sin(2*q2 + q3))/2 + (dq1*l2*l3*m5*sin(2*q2 + q3))/2 + (dq1*l2*l3*m6*sin(2*q2 + q3))/2 + (dq1*l2*lc3*m3*sin(2*q2 + q3))/2 - (dc6*dq1*l2*m6*cos(2*q2 + q3 + q4 - q5))/4 + (dc6*dq1*l3*m6*cos(2*q2 + 2*q3 + q4 + q5))/2 - (d5*dq1*l2*m6*cos(2*q2 + q3 + q4))/2 - (dc5*dq1*l2*m5*cos(2*q2 + q3 + q4))/2 - (dc6*dq1*l2*m6*cos(q3 + q4 - q5))/4 - (d5*dq1*l2*m6*cos(q3 + q4))/2 - (dc5*dq1*l2*m5*cos(q3 + q4))/2 - (dc6*dq1*l3*m6*cos(2*q2 + 2*q3 + q4 - q5))/2 + (d5*dc6*dq1*m6*sin(2*q2 + 2*q3 + 2*q4 + q5))/2 - d5*dq1*l3*m6*cos(2*q2 + 2*q3 + q4) - dc5*dq1*l3*m5*cos(2*q2 + 2*q3 + q4) + (dc6*dq1*l2*m6*cos(2*q2 + q3 + q4 + q5))/4 + (dq1*l2*l3*m4*sin(q3))/2 + (dq1*l2*l3*m5*sin(q3))/2 + (dq1*l2*l3*m6*sin(q3))/2 + (dq1*l2*lc3*m3*sin(q3))/2;
C(3,2) = dq2*l2*(l3*m4*sin(q3) + l3*m5*sin(q3) + l3*m6*sin(q3) + lc3*m3*sin(q3) - d5*m6*cos(q3 + q4) - dc5*m5*cos(q3 + q4) - dc6*m6*cos(q3)*sin(q4)*sin(q5) - dc6*m6*cos(q4)*sin(q3)*sin(q5));
C(3,3) = 0;
C(3,4) = l3*(2*dq2 + 2*dq3 + dq4)*(d5*m6*cos(q4) + dc5*m5*cos(q4) + dc6*m6*sin(q4)*sin(q5));
C(3,5) = -dc6*m6*(dq2*l3*cos(q4 - q5) - d5*dq1*sin(q2 + q3 + q4 - q5) - (dc6*dq1*sin(q2 + q3 + q4 - 2*q5))/2 - (dc6*dq1*sin(q2 + q3 + q4 + 2*q5))/2 - d5*dq5*sin(q5) + dq3*l3*cos(q4 - q5) + dq4*l3*cos(q4 - q5) - (dq5*l3*cos(q4 - q5))/2 + dq1*l3*cos(q2 + q3 + q5) + dc6*dq1*sin(q2 + q3 + q4) - dc6*dq2*sin(2*q5) - dc6*dq3*sin(2*q5) - dc6*dq4*sin(2*q5) - dq1*l3*cos(q2 + q3 - q5) + d5*dq1*sin(q2 + q3 + q4 + q5) + dq2*l3*cos(q4 + q5) + dq3*l3*cos(q4 + q5) + dq4*l3*cos(q4 + q5) + (dq5*l3*cos(q4 + q5))/2);
C(3,6) = 0;

C(4,1) = (dc6^2*dq1*m6*sin(2*q2 + 2*q3 + 2*q4))/4 - (dc6^2*dq1*m6*sin(2*q2 + 2*q3 + 2*q4 + 2*q5))/8 - (d5^2*dq1*m6*sin(2*q2 + 2*q3 + 2*q4))/2 - (dc5^2*dq1*m5*sin(2*q2 + 2*q3 + 2*q4))/2 - (dc6^2*dq1*m6*sin(2*q2 + 2*q3 + 2*q4 - 2*q5))/8 - (dc6*dq1*l3*m6*cos(q4 - q5))/4 - (d5*dc6*dq1*m6*sin(2*q2 + 2*q3 + 2*q4 - q5))/2 + (dc6*dq1*l2*m6*cos(q3 + q4 + q5))/4 - (dc6*dq1*l2*m6*cos(2*q2 + q3 + q4 - q5))/4 + (dc6*dq1*l3*m6*cos(2*q2 + 2*q3 + q4 + q5))/4 - (d5*dq1*l2*m6*cos(2*q2 + q3 + q4))/2 - (dc5*dq1*l2*m5*cos(2*q2 + q3 + q4))/2 - (dc6*dq1*l2*m6*cos(q3 + q4 - q5))/4 - (d5*dq1*l2*m6*cos(q3 + q4))/2 - (dc5*dq1*l2*m5*cos(q3 + q4))/2 + (dc6*dq1*l3*m6*cos(q4 + q5))/4 - (dc6*dq1*l3*m6*cos(2*q2 + 2*q3 + q4 - q5))/4 + (d5*dc6*dq1*m6*sin(2*q2 + 2*q3 + 2*q4 + q5))/2 - (d5*dq1*l3*m6*cos(q4))/2 - (d5*dq1*l3*m6*cos(2*q2 + 2*q3 + q4))/2 - (dc5*dq1*l3*m5*cos(q4))/2 - (dc5*dq1*l3*m5*cos(2*q2 + 2*q3 + q4))/2 + (dc6*dq1*l2*m6*cos(2*q2 + q3 + q4 + q5))/4;
C(4,2) = - dq2*(l2*cos(q3 + q4) + l3*cos(q4))*(d5*m6 + dc5*m5) - dc6*dq2*l3*m6*sin(q4)*sin(q5) - dc6*dq2*l2*m6*cos(q3)*sin(q4)*sin(q5) - dc6*dq2*l2*m6*cos(q4)*sin(q3)*sin(q5);
C(4,3) = -l3*(2*dq2 + dq3)*(d5*m6*cos(q4) + dc5*m5*cos(q4) + dc6*m6*sin(q4)*sin(q5));
C(4,4) = 0;
C(4,5) = (dc6*m6*(2*d5*dq5*sin(q5) + 2*d5*dq1*sin(q2 + q3 + q4 - q5) + dc6*dq1*sin(q2 + q3 + q4 - 2*q5) + dc6*dq1*sin(q2 + q3 + q4 + 2*q5) - 2*dc6*dq1*sin(q2 + q3 + q4) + 2*dc6*dq2*sin(2*q5) + 2*dc6*dq3*sin(2*q5) + 2*dc6*dq4*sin(2*q5) - 2*d5*dq1*sin(q2 + q3 + q4 + q5)))/2;
C(4,6) = 0;

C(5,1) = (dc6*dq1*m6*(2*dc6*sin(2*q5) + 2*l2*cos(2*q2 + q3 + q4 - q5) + 2*l3*cos(2*q2 + 2*q3 + q4 + q5) + 2*l2*cos(q3 + q4 - q5) + 2*l3*cos(q4 + q5) + 2*l3*cos(2*q2 + 2*q3 + q4 - q5) + 2*d5*sin(2*q2 + 2*q3 + 2*q4 + q5) + 8*d4*sin(q5) + 2*l2*cos(2*q2 + q3 + q4 + q5) + 2*l3*cos(q4 - q5) + 2*d5*sin(2*q2 + 2*q3 + 2*q4 - q5) + dc6*sin(2*q2 + 2*q3 + 2*q4 - 2*q5) - dc6*sin(2*q2 + 2*q3 + 2*q4 + 2*q5) + 2*l2*cos(q3 + q4 + q5)))/8;
C(5,2) = (dc6*m6*(dq2*l3*cos(q4 - q5) - dc6*dq1*sin(q2 + q3 + q4 - 2*q5) - dc6*dq1*sin(q2 + q3 + q4 + 2*q5) - 2*dq1*l2*cos(q2 - q5) - 2*d5*dq1*sin(q2 + q3 + q4 - q5) + 2*dq1*l3*cos(q2 + q3 + q5) + dq2*l2*cos(q3 + q4 + q5) + 2*dc6*dq1*sin(q2 + q3 + q4) - dc6*dq2*sin(2*q5) - 2*dq1*l3*cos(q2 + q3 - q5) + dq2*l2*cos(q3 + q4 - q5) + 2*d5*dq1*sin(q2 + q3 + q4 + q5) + 2*dq1*l2*cos(q2 + q5) + dq2*l3*cos(q4 + q5)))/2;
C(5,3) = (dc6*m6*(2*dq2*l3*cos(q4 - q5) - dc6*dq1*sin(q2 + q3 + q4 - 2*q5) - dc6*dq1*sin(q2 + q3 + q4 + 2*q5) - 2*d5*dq1*sin(q2 + q3 + q4 - q5) + dq3*l3*cos(q4 - q5) + 2*dq1*l3*cos(q2 + q3 + q5) + 2*dc6*dq1*sin(q2 + q3 + q4) - 2*dc6*dq2*sin(2*q5) - dc6*dq3*sin(2*q5) - 2*dq1*l3*cos(q2 + q3 - q5) + 2*d5*dq1*sin(q2 + q3 + q4 + q5) + 2*dq2*l3*cos(q4 + q5) + dq3*l3*cos(q4 + q5)))/2;
C(5,4) = -(dc6*m6*(2*d5*dq1*sin(q2 + q3 + q4 - q5) + dc6*dq1*sin(q2 + q3 + q4 - 2*q5) + dc6*dq1*sin(q2 + q3 + q4 + 2*q5) - 2*dc6*dq1*sin(q2 + q3 + q4) + 2*dc6*dq2*sin(2*q5) + 2*dc6*dq3*sin(2*q5) + dc6*dq4*sin(2*q5) - 2*d5*dq1*sin(q2 + q3 + q4 + q5)))/2;
C(5,5) = 0;
C(5,6) = 0;

C(6,1) = 0;
C(6,2) = 0;
C(6,3) = 0;
C(6,4) = 0;
C(6,5) = 0;
C(6,6) = 0;



% Matriz de Gravedad G: 
G = zeros(6,1);

G(1,1) = 0;

G(2,1) = l2*m3*cos(q2) + l2*m4*cos(q2) + l2*m5*cos(q2) + l2*m6*cos(q2) + lc2*m2*cos(q2) + (dc6*m6*sin(q2 + q3 + q4 - q5))/2 + d5*m6*sin(q2 + q3 + q4) + dc5*m5*sin(q2 + q3 + q4) - (dc6*m6*sin(q2 + q3 + q4 + q5))/2 + l3*m4*cos(q2 + q3) + l3*m5*cos(q2 + q3) + l3*m6*cos(q2 + q3) + lc3*m3*cos(q2 + q3);

G(3,1) = (dc6*m6*sin(q2 + q3 + q4 - q5))/2 + d5*m6*sin(q2 + q3 + q4) + dc5*m5*sin(q2 + q3 + q4) - (dc6*m6*sin(q2 + q3 + q4 + q5))/2 + l3*m4*cos(q2 + q3) + l3*m5*cos(q2 + q3) + l3*m6*cos(q2 + q3) + lc3*m3*cos(q2 + q3);

G(4,1) = (dc6*m6*sin(q2 + q3 + q4 - q5))/2 + d5*m6*sin(q2 + q3 + q4) + dc5*m5*sin(q2 + q3 + q4) - (dc6*m6*sin(q2 + q3 + q4 + q5))/2;

G(5,1) = -(dc6*m6*(sin(q2 + q3 + q4 + q5) + sin(q2 + q3 + q4 - q5)))/2;

G(6,1) = 0;


robot_din = struct('D',D,'C',C,'G',G,'g',9.81);

%busInfo = Simulink.Bus.createObject(robot_dyn);

== matlab function control_pos_6dof_conMI/Controlador/Controlador de posición ==
  data: robot_din input; A0 input; A1 input; tau_R output; q_ref input; dq_ref input; ddq_ref input; q input; dq input
function tau_R = fcn(robot_din,A0,A1,q_ref,dq_ref,ddq_ref,q,dq)

D = robot_din.D;
C = robot_din.C;
G = robot_din.G;
g = robot_din.g;

tau_R = D*(ddq_ref+A1.*dq_ref+A0.*q_ref-A1.*dq-A0.*q)+(C*dq+G*g);

== matlab function control_pos_6dof_conMI/Actuadores (Motores de inducción)/MI4 + PBC Torque Controller/Calculo de Potencia eléctrica/Blondel-Park-u_Sab ==
  data: BPU1 input; BPU2 input; U1 output; U2 output; U3 output
function [U1,U2,U3]   = fcn(BPU1,BPU2)

U1=BPU1;
U2=-BPU1/2-sqrt(3)*BPU2/2;
U3=-BPU1/2+sqrt(3)*BPU2/2;

== matlab function control_pos_6dof_conMI/Actuadores (Motores de inducción)/MI1 + PBC Torque Controller/Controlador PBC/Corrientes y Flujos deseados/Corrientes//Flujos deseados ==
  data: MI_motor_params input; w_R input; i_Sref output size=[2 1]; psi_Rref input size=[2,1]; tau_Rref input; psi_Rmagref input; dpsi_Rmagref input; dpsi_Rref output size=[2,1]
function [i_Sref,dpsi_Rref] = fcn(MI_motor_params,w_R,psi_Rref,tau_Rref,psi_Rmagref,dpsi_Rmagref)

R_R = MI_motor_params.elecparams.R_R;
L_R = MI_motor_params.elecparams.L_R;
M = MI_motor_params.elecparams.M;
n_p = MI_motor_params.elecparams.n_p;

psi_Raref = psi_Rref(1);
psi_Rbref = psi_Rref(2);

i_Saref =  - L_R/(M*n_p*psi_Rmagref^2)*tau_Rref*psi_Rbref + 1/M*psi_Raref + L_R/(R_R*M)*dpsi_Rmagref/psi_Rmagref*psi_Raref;
i_Sbref =  + L_R/(M*n_p*psi_Rmagref^2)*tau_Rref*psi_Raref + 1/M*psi_Rbref + L_R/(R_R*M)*dpsi_Rmagref/psi_Rmagref*psi_Rbref;

i_Sref = [i_Saref;i_Sbref];

dpsi_Raref = - (n_p*w_R + R_R/(n_p*psi_Rmagref^2)*tau_Rref)*psi_Rbref + dpsi_Rmagref/psi_Rmagref*psi_Raref;
dpsi_Rbref = + (n_p*w_R + R_R/(n_p*psi_Rmagref^2)*tau_Rref)*psi_Raref + dpsi_Rmagref/psi_Rmagref*psi_Rbref;

dpsi_Rref = [dpsi_Raref;dpsi_Rbref];

== matlab function control_pos_6dof_conMI/Actuadores (Motores de inducción)/MI1 + PBC Torque Controller/Controlador PBC/Ley de control/K_iS ==
  data: MI_motor_params input; w_R input; epsilon input; K_iS output
function K_iS = fcn(MI_motor_params,w_R,epsilon)

R_R = MI_motor_params.elecparams.R_R;
M = MI_motor_params.elecparams.M;
L_R = MI_motor_params.elecparams.L_R;
n_p = MI_motor_params.elecparams.n_p;


K_iS = M^2*L_R*n_p^2*w_R^2/(epsilon*4*R_R);

== matlab function control_pos_6dof_conMI/Actuadores (Motores de inducción)/MI1 + PBC Torque Controller/Controlador PBC/Ley de control/Ley de control ==
  data: MI_motor_params input; i_Sref input size=[2,1]; d_iSref input size=[2,1]; U_S output size=[2 1]; psi_Rref input size=[2,1]; w_R input; e_Is input; KI_s input
function U_S = fcn(MI_motor_params,i_Sref,d_iSref,psi_Rref,w_R,e_Is,KI_s)

R_R = MI_motor_params.elecparams.R_R;
L_R = MI_motor_params.elecparams.L_R;
M = MI_motor_params.elecparams.M;
n_p = MI_motor_params.elecparams.n_p;

sigma = MI_motor_params.elecparams.sigma;
gamma = MI_motor_params.elecparams.gamma;

dI_Saref = d_iSref(1);
dI_Sbref = d_iSref(2);

I_Saref = i_Sref(1);
I_Sbref = i_Sref(2);

psi_Raref = psi_Rref(1);
psi_Rbref = psi_Rref(2);

e_ISa = e_Is(1);
e_ISb = e_Is(2);

U_Sa = sigma*dI_Saref - n_p*M/L_R*w_R*psi_Rbref + sigma*gamma*I_Saref - R_R*M/L_R^2*psi_Raref - KI_s*e_ISa;
U_Sb = sigma*dI_Sbref + n_p*M/L_R*w_R*psi_Raref + sigma*gamma*I_Sbref - R_R*M/L_R^2*psi_Rbref - KI_s*e_ISb;

U_S = [U_Sa;U_Sb];

== matlab function control_pos_6dof_conMI/Actuadores (Motores de inducción)/MI1 + PBC Torque Controller/Calculo de Potencia eléctrica/Blondel-Park-i_Sab ==
  data: BPU1 input; BPU2 input; U1 output; U2 output; U3 output
function [U1,U2,U3]   = fcn(BPU1,BPU2)

U1=BPU1;
U2=-BPU1/2-sqrt(3)*BPU2/2;
U3=-BPU1/2+sqrt(3)*BPU2/2;

== matlab function control_pos_6dof_conMI/Actuadores (Motores de inducción)/MI1 + PBC Torque Controller/Calculo de Potencia eléctrica/Blondel-Park-u_Sab ==
  data: BPU1 input; BPU2 input; U1 output; U2 output; U3 output
function [U1,U2,U3]   = fcn(BPU1,BPU2)

U1=BPU1;
U2=-BPU1/2-sqrt(3)*BPU2/2;
U3=-BPU1/2+sqrt(3)*BPU2/2;

== matlab function control_pos_6dof_conMI/Actuadores (Motores de inducción)/MI2 + PBC Torque Controller/Calculo de Potencia eléctrica/Blondel-Park-i_Sab ==
  data: BPU1 input; BPU2 input; U1 output; U2 output; U3 output
function [U1,U2,U3]   = fcn(BPU1,BPU2)

U1=BPU1;
U2=-BPU1/2-sqrt(3)*BPU2/2;
U3=-BPU1/2+sqrt(3)*BPU2/2;

== matlab function control_pos_6dof_conMI/Inicializar posición de robot manipulador/dq_init/q1/Polinomio 7mo orden dq ==
  data: t input; q0 input; qpol output; vpol output; apol output; jpol output; q1 input; t0 input; t1 input
function [qpol,vpol,apol,jpol] = fcn(t,q0,q1,t0,t1)


% t,q0,q1,v0,v1,ac0,ac1,j0,j1,t0,t1)
%Trayectoria de referencia

% q0 = 0;
% q1 = 0;

v0 = 0;
v1 = 0;

ac0 = 0;
ac1 = 0;

j0 = 0;
j1 = 0;

% t0 = 0;
% t1 = pi/4;

% Coeficientes de un polinomio de 7mo grado

h = q1 - q0;
T = t1 - t0;

a = zeros(7+1,1);

a(1) = q0;
a(2) = v0;
a(3) = ac0/2;
a(4) = j0/6;
a(5) = (210*h-T*((30*ac0-15*ac1)*T+(4*j0+j1)*T^2+120*v0+90*v1))/(6*T^4);
a(6) = (-168*h-T*((20*ac0-14*ac1)*T+(2*j0+j1)*T^2+90*v0+78*v1))/(2*T^5);
a(7) = (420*h-T*((45*ac0-39*ac1)*T+(4*j0+3*j1)*T^2+216*v0+204*v1))/(6*T^6);
a(8) = (-120*h-T*((12*ac0-12*ac1)*T+(j0+j1)*T^2+60*v0+60*v1))/(6*T^7);

qa = flip(a')';
va = polyder(qa')';
aa = polyder(va')';
ja = polyder(aa')';


if t>=t0 && t<t1
    qpol = polyval(qa,t-t0);
    vpol = polyval(va,t-t0);
    apol = polyval(aa,t-t0);
    jpol = polyval(ja,t-t0);
elseif t>=t1
    qpol = polyval(qa,T);
    vpol = polyval(va,T);
    apol = polyval(aa,T);
    jpol = polyval(ja,T);
else
    qpol = q0;
    vpol = v0;
    apol = ac0;
    jpol = j0;
end

== matlab function control_pos_6dof_conMI/Actuadores (Motores de inducción)/MI2 + PBC Torque Controller/Calculo de Potencia eléctrica/Blondel-Park-u_Sab ==
  data: BPU1 input; BPU2 input; U1 output; U2 output; U3 output
function [U1,U2,U3]   = fcn(BPU1,BPU2)

U1=BPU1;
U2=-BPU1/2-sqrt(3)*BPU2/2;
U3=-BPU1/2+sqrt(3)*BPU2/2;

== matlab function control_pos_6dof_conMI/Actuadores (Motores de inducción)/MI2 + PBC Torque Controller/Controlador PBC/Corrientes y Flujos deseados/Corrientes//Flujos deseados ==
  data: MI_motor_params input; w_R input; i_Sref output size=[2 1]; psi_Rref input size=[2,1]; tau_Rref input; psi_Rmagref input; dpsi_Rmagref input; dpsi_Rref output size=[2,1]
function [i_Sref,dpsi_Rref] = fcn(MI_motor_params,w_R,psi_Rref,tau_Rref,psi_Rmagref,dpsi_Rmagref)

R_R = MI_motor_params.elecparams.R_R;
L_R = MI_motor_params.elecparams.L_R;
M = MI_motor_params.elecparams.M;
n_p = MI_motor_params.elecparams.n_p;

psi_Raref = psi_Rref(1);
psi_Rbref = psi_Rref(2);

i_Saref =  - L_R/(M*n_p*psi_Rmagref^2)*tau_Rref*psi_Rbref + 1/M*psi_Raref + L_R/(R_R*M)*dpsi_Rmagref/psi_Rmagref*psi_Raref;
i_Sbref =  + L_R/(M*n_p*psi_Rmagref^2)*tau_Rref*psi_Raref + 1/M*psi_Rbref + L_R/(R_R*M)*dpsi_Rmagref/psi_Rmagref*psi_Rbref;

i_Sref = [i_Saref;i_Sbref];

dpsi_Raref = - (n_p*w_R + R_R/(n_p*psi_Rmagref^2)*tau_Rref)*psi_Rbref + dpsi_Rmagref/psi_Rmagref*psi_Raref;
dpsi_Rbref = + (n_p*w_R + R_R/(n_p*psi_Rmagref^2)*tau_Rref)*psi_Raref + dpsi_Rmagref/psi_Rmagref*psi_Rbref;

dpsi_Rref = [dpsi_Raref;dpsi_Rbref];

== matlab function control_pos_6dof_conMI/Actuadores (Motores de inducción)/MI1 + PBC Torque Controller/Controlador PBC/derivada Corrientes deseadas/derivada Corrientes deseadas ==
  data: MI_motor_params input; d_iSref output size=[2 1]; psi_Rref input size=[2,1]; dpsi_Rref input size=[2,1]; psi_Rmagref input; dpsi_Rmagref input; ddpsi_Rmagref input; tau_Rref input; dtau_Rref input
function d_iSref = fcn(MI_motor_params,psi_Rref,dpsi_Rref,psi_Rmagref,dpsi_Rmagref,ddpsi_Rmagref,tau_Rref,dtau_Rref)

R_R = MI_motor_params.elecparams.R_R;
L_R = MI_motor_params.elecparams.L_R;
M = MI_motor_params.elecparams.M;
n_p = MI_motor_params.elecparams.n_p;

dpsi_Raref = dpsi_Rref(1);
dpsi_Rbref = dpsi_Rref(2);

psi_Raref = psi_Rref(1);
psi_Rbref = psi_Rref(2);

dI_Saref = L_R/(M*n_p)*(- ((dtau_Rref-2*tau_Rref*dpsi_Rmagref)/psi_Rmagref)*psi_Rbref - tau_Rref/psi_Rmagref^2*dpsi_Rbref) + dpsi_Raref/M ...
         + L_R/(R_R*M)*(((ddpsi_Rmagref*psi_Rmagref-dpsi_Rmagref^2)/psi_Rmagref^2)*psi_Raref + dpsi_Rmagref/psi_Rmagref*dpsi_Raref);

dI_Sbref = L_R/(M*n_p)*(+ ((dtau_Rref-2*tau_Rref*dpsi_Rmagref)/psi_Rmagref)*psi_Raref + tau_Rref/psi_Rmagref^2*dpsi_Raref) + dpsi_Rbref/M ...
         + L_R/(R_R*M)*(((ddpsi_Rmagref*psi_Rmagref-dpsi_Rmagref^2)/psi_Rmagref^2)*psi_Rbref + dpsi_Rmagref/psi_Rmagref*dpsi_Rbref);

d_iSref = [dI_Saref;dI_Sbref];

== matlab function control_pos_6dof_conMI/Actuadores (Motores de inducción)/MI1 + PBC Torque Controller/Modelo MI (Subsistema eléctrico)/Modelo Motor de inducción (Subsistema eléctrico) ==
  data: MI_motor_params input; di_Sab output double size=[2 1]; dpsi_Rab output double size=[2 1]; u_Sab input double size=[2 1]; i_Sab input double size=[2 1]; psi_Rab input double size=[2 1]; w_R input double size=1; tau_R output size=1; tau_L input
function [di_Sab,dpsi_Rab,tau_R] = fcn(MI_motor_params,u_Sab,i_Sab,psi_Rab,w_R,tau_L)

R_S = MI_motor_params.elecparams.R_S;
R_R = MI_motor_params.elecparams.R_R;
L_S = MI_motor_params.elecparams.L_S;
L_R = MI_motor_params.elecparams.L_R;
M = MI_motor_params.elecparams.M;
n_p = MI_motor_params.elecparams.n_p;

J = MI_motor_params.mechparams.J;
b = MI_motor_params.mechparams.b;

sigma = MI_motor_params.elecparams.sigma;
gamma = MI_motor_params.elecparams.gamma;

u_sa = u_Sab(1);
u_sb = u_Sab(2);

i_sa = i_Sab(1);
i_sb = i_Sab(2);

psi_ra = psi_Rab(1);
psi_rb = psi_Rab(2);

tau_R = 3/2*n_p*M/L_R*(i_sb*psi_ra-i_sa*psi_rb);

x = [i_sa;i_sb;psi_ra;psi_rb];

A = [-gamma      , 0            , (M*R_R)/(sigma*L_R^2)    , (n_p*M)/(sigma*L_R)*w_R ;
     0           , -gamma       , -(n_p*M)/(sigma*L_R)*w_R , (M*R_R)/(sigma*L_R^2)   ; 
     (R_R*M)/L_R , 0            , -R_R/L_R                 , -n_p*w_R                ;
     0           , (R_R*M)/L_R  , n_p*w_R                  , -R_R/L_R                ];

B = [1/sigma , 0       ;
     0       , 1/sigma ;
     0       , 0       ;
     0       , 0       ];

dx = A*x + B*[u_sa;u_sb];

di_Sab = dx(1:2);
dpsi_Rab = dx(3:4);

%Subsistema mecanico
%dw_R = (1/J)*tau_R - (b/J)*w_R - (1/J)*tau_L;

== matlab function control_pos_6dof_conMI/Actuadores (Motores de inducción)/MI1 + PBC Torque Controller/Modelo MI (Subsistema eléctrico)/ab//dq ==
  data: psi_ra input; psi_Rmag output; psi_rb input; rho output
function [psi_Rmag,rho] = fcn(psi_ra,psi_rb)

psi_Rmag = sqrt(psi_ra^2+psi_rb^2);
rho = atan2(psi_rb,psi_ra);

== matlab function control_pos_6dof_conMI/Actuadores (Motores de inducción)/MI2 + PBC Torque Controller/Controlador PBC/Ley de control/K_iS ==
  data: MI_motor_params input; w_R input; epsilon input; K_iS output
function K_iS = fcn(MI_motor_params,w_R,epsilon)

R_R = MI_motor_params.elecparams.R_R;
M = MI_motor_params.elecparams.M;
L_R = MI_motor_params.elecparams.L_R;
n_p = MI_motor_params.elecparams.n_p;


K_iS = M^2*L_R*n_p^2*w_R^2/(epsilon*4*R_R);

== matlab function control_pos_6dof_conMI/Actuadores (Motores de inducción)/MI2 + PBC Torque Controller/Controlador PBC/Ley de control/Ley de control ==
  data: MI_motor_params input; i_Sref input size=[2,1]; d_iSref input size=[2,1]; U_S output size=[2 1]; psi_Rref input size=[2,1]; w_R input; e_Is input; KI_s input
function U_S = fcn(MI_motor_params,i_Sref,d_iSref,psi_Rref,w_R,e_Is,KI_s)

R_R = MI_motor_params.elecparams.R_R;
L_R = MI_motor_params.elecparams.L_R;
M = MI_motor_params.elecparams.M;
n_p = MI_motor_params.elecparams.n_p;

sigma = MI_motor_params.elecparams.sigma;
gamma = MI_motor_params.elecparams.gamma;

dI_Saref = d_iSref(1);
dI_Sbref = d_iSref(2);

I_Saref = i_Sref(1);
I_Sbref = i_Sref(2);

psi_Raref = psi_Rref(1);
psi_Rbref = psi_Rref(2);

e_ISa = e_Is(1);
e_ISb = e_Is(2);

U_Sa = sigma*dI_Saref - n_p*M/L_R*w_R*psi_Rbref + sigma*gamma*I_Saref - R_R*M/L_R^2*psi_Raref - KI_s*e_ISa;
U_Sb = sigma*dI_Sbref + n_p*M/L_R*w_R*psi_Raref + sigma*gamma*I_Sbref - R_R*M/L_R^2*psi_Rbref - KI_s*e_ISb;

U_S = [U_Sa;U_Sb];

== matlab function control_pos_6dof_conMI/Actuadores (Motores de inducción)/MI2 + PBC Torque Controller/Controlador PBC/derivada Corrientes deseadas/derivada Corrientes deseadas ==
  data: MI_motor_params input; d_iSref output size=[2 1]; psi_Rref input size=[2,1]; dpsi_Rref input size=[2,1]; psi_Rmagref input; dpsi_Rmagref input; ddpsi_Rmagref input; tau_Rref input; dtau_Rref input
function d_iSref = fcn(MI_motor_params,psi_Rref,dpsi_Rref,psi_Rmagref,dpsi_Rmagref,ddpsi_Rmagref,tau_Rref,dtau_Rref)

R_R = MI_motor_params.elecparams.R_R;
L_R = MI_motor_params.elecparams.L_R;
M = MI_motor_params.elecparams.M;
n_p = MI_motor_params.elecparams.n_p;

dpsi_Raref = dpsi_Rref(1);
dpsi_Rbref = dpsi_Rref(2);

psi_Raref = psi_Rref(1);
psi_Rbref = psi_Rref(2);

dI_Saref = L_R/(M*n_p)*(- ((dtau_Rref-2*tau_Rref*dpsi_Rmagref)/psi_Rmagref)*psi_Rbref - tau_Rref/psi_Rmagref^2*dpsi_Rbref) + dpsi_Raref/M ...
         + L_R/(R_R*M)*(((ddpsi_Rmagref*psi_Rmagref-dpsi_Rmagref^2)/psi_Rmagref^2)*psi_Raref + dpsi_Rmagref/psi_Rmagref*dpsi_Raref);

dI_Sbref = L_R/(M*n_p)*(+ ((dtau_Rref-2*tau_Rref*dpsi_Rmagref)/psi_Rmagref)*psi_Raref + tau_Rref/psi_Rmagref^2*dpsi_Raref) + dpsi_Rbref/M ...
         + L_R/(R_R*M)*(((ddpsi_Rmagref*psi_Rmagref-dpsi_Rmagref^2)/psi_Rmagref^2)*psi_Rbref + dpsi_Rmagref/psi_Rmagref*dpsi_Rbref);

d_iSref = [dI_Saref;dI_Sbref];

== matlab function control_pos_6dof_conMI/Actuadores (Motores de inducción)/MI2 + PBC Torque Controller/Modelo MI (Subsistema eléctrico)/Modelo Motor de inducción (Subsistema eléctrico) ==
  data: MI_motor_params input; di_Sab output double size=[2 1]; dpsi_Rab output double size=[2 1]; u_Sab input double size=[2 1]; i_Sab input double size=[2 1]; psi_Rab input double size=[2 1]; w_R input double size=1; tau_R output size=1; tau_L input
function [di_Sab,dpsi_Rab,tau_R] = fcn(MI_motor_params,u_Sab,i_Sab,psi_Rab,w_R,tau_L)

R_S = MI_motor_params.elecparams.R_S;
R_R = MI_motor_params.elecparams.R_R;
L_S = MI_motor_params.elecparams.L_S;
L_R = MI_motor_params.elecparams.L_R;
M = MI_motor_params.elecparams.M;
n_p = MI_motor_params.elecparams.n_p;

J = MI_motor_params.mechparams.J;
b = MI_motor_params.mechparams.b;

sigma = MI_motor_params.elecparams.sigma;
gamma = MI_motor_params.elecparams.gamma;

u_sa = u_Sab(1);
u_sb = u_Sab(2);

i_sa = i_Sab(1);
i_sb = i_Sab(2);

psi_ra = psi_Rab(1);
psi_rb = psi_Rab(2);

tau_R = 3/2*n_p*M/L_R*(i_sb*psi_ra-i_sa*psi_rb);

x = [i_sa;i_sb;psi_ra;psi_rb];

A = [-gamma      , 0            , (M*R_R)/(sigma*L_R^2)    , (n_p*M)/(sigma*L_R)*w_R ;
     0           , -gamma       , -(n_p*M)/(sigma*L_R)*w_R , (M*R_R)/(sigma*L_R^2)   ; 
     (R_R*M)/L_R , 0            , -R_R/L_R                 , -n_p*w_R                ;
     0           , (R_R*M)/L_R  , n_p*w_R                  , -R_R/L_R                ];

B = [1/sigma , 0       ;
     0       , 1/sigma ;
     0       , 0       ;
     0       , 0       ];

dx = A*x + B*[u_sa;u_sb];

di_Sab = dx(1:2);
dpsi_Rab = dx(3:4);

%Subsistema mecanico
%dw_R = (1/J)*tau_R - (b/J)*w_R - (1/J)*tau_L;

== matlab function control_pos_6dof_conMI/Actuadores (Motores de inducción)/MI2 + PBC Torque Controller/Modelo MI (Subsistema eléctrico)/ab//dq ==
  data: psi_ra input; psi_Rmag output; psi_rb input; rho output
function [psi_Rmag,rho] = fcn(psi_ra,psi_rb)

psi_Rmag = sqrt(psi_ra^2+psi_rb^2);
rho = atan2(psi_rb,psi_ra);

== matlab function control_pos_6dof_conMI/Actuadores (Motores de inducción)/MI6 + PBC Torque Controller/Calculo de Potencia eléctrica/Blondel-Park-i_Sab ==
  data: BPU1 input; BPU2 input; U1 output; U2 output; U3 output
function [U1,U2,U3]   = fcn(BPU1,BPU2)

U1=BPU1;
U2=-BPU1/2-sqrt(3)*BPU2/2;
U3=-BPU1/2+sqrt(3)*BPU2/2;

== matlab function control_pos_6dof_conMI/Actuadores (Motores de inducción)/MI6 + PBC Torque Controller/Calculo de Potencia eléctrica/Blondel-Park-u_Sab ==
  data: BPU1 input; BPU2 input; U1 output; U2 output; U3 output
function [U1,U2,U3]   = fcn(BPU1,BPU2)

U1=BPU1;
U2=-BPU1/2-sqrt(3)*BPU2/2;
U3=-BPU1/2+sqrt(3)*BPU2/2;
